simulink model "PMSMwithPSWM"  (R2018a)
settings: Solver=FixedStepDiscrete  StartTime=0.0  StopTime=4  FixedStep=1e-6  RelTol=1e-3
libraries: powerlib x28, simulink x6, powerlib_meascontrol x1
settings Model: Creator=user  LastModifiedBy=Administrator

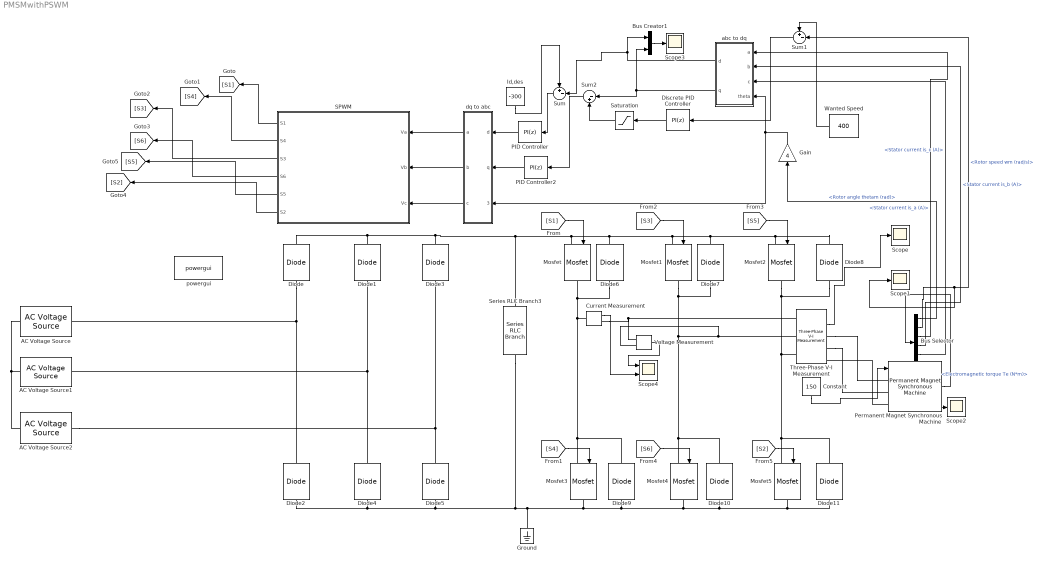
== system PMSMwithPSWM ==
  AC Voltage Source : powerlib/Electrical Sources/AC Voltage Source  Amplitude=230  Phase=0  Frequency=50  SampleTime=0  Measurements=None  BusType=swing  Pref=10e3  Qref=0  Qmin=-inf  Qmax=+inf
  AC Voltage Source1 : powerlib/Electrical Sources/AC Voltage Source  Amplitude=230  Phase=120  Frequency=50  SampleTime=0  Measurements=None  BusType=swing  Pref=10e3  Qref=0  Qmin=-inf  Qmax=+inf
  AC Voltage Source2 : powerlib/Electrical Sources/AC Voltage Source  Amplitude=230  Phase=240  Frequency=50  SampleTime=0  Measurements=None  BusType=swing  Pref=10e3  Qref=0  Qmin=-inf  Qmax=+inf
  Bus Creator1 : BusCreator  Inputs=2
  Bus Selector : BusSelector  OutputSignals=Rotor angle thetam (rad),Rotor speed wm (rad/s),Stator current is_a (A),Stator current is_b (A),Stator current is_c (A),Electromagnetic torque Te (N*m)
  Constant : Constant  Value=150
  Current Measurement : powerlib/Measurements/Current Measurement  PhasorSimulation=off  OutputType=Complex  PSBequivalent=0
  Diode{,1..5} (6 alike) : powerlib/Power Electronics/Diode  Ron=0.02  Lon=0  Vf=0.8  IC=0  UseSnubber=0  Rs=500  Cs=250e-9  Measurements=off
  Diode{6..11} (6 alike) : powerlib/Power Electronics/Diode  Ron=0.001  Lon=0  Vf=0.8  IC=0  UseSnubber=0  Rs=500  Cs=250e-9  Measurements=off
  Discrete PID Controller : simulink/Continuous/PID Controller  Controller=PI  TimeDomain=Discrete-time  SampleTime=-1  IntegratorMethod=Forward Euler  FilterMethod=Forward Euler  Form=Parallel  UseFilter=on  ControllerParametersSource=internal  P=800  I=1  D=0  N=100  InitialConditionSource=internal  InitialConditionForIntegrator=0  InitialConditionForFilter=0  ExternalReset=none  LimitOutput=off  UpperSaturationLimit=inf  LowerSaturationLimit=-inf  LinearizeAsGain=off  AntiWindupMode=none  Kb=1  TrackingMode=off  Kt=1  PParamMin=[]  PParamMax=[]  IParamMin=[]  IParamMax=[]  DParamMin=[]  DParamMax=[]  NParamMin=[]  NParamMax=[]  KbParamMin=[]  KbParamMax=[]  KtParamMin=[]  KtParamMax=[]  POutMin=[]  POutMax=[]  IOutMin=[]  IOutMax=[]  DOutMin=[]  DOutMax=[]  NOutMin=[]  NOutMax=[]  KbOutMin=[]  KbOutMax=[]  KtOutMin=[]  KtOutMax=[]  IntegratorOutMin=[]  IntegratorOutMax=[]  FilterOutMin=[]  FilterOutMax=[]  SumOutMin=[]  SumOutMax=[]  SumI1OutMin=[]  SumI1OutMax=[]  SumI2OutMin=[]  SumI2OutMax=[]  SumI3OutMin=[]  SumI3OutMax=[]  SumDOutMin=[]  SumDOutMax=[]  SaturationOutMin=[]  SaturationOutMax=[]  IntegratorContinuousStateAttributes=''  IntegratorStateMustResolveToSignalObject=off  IntegratorRTWStateStorageClass=Auto  FilterContinuousStateAttributes=''  FilterStateMustResolveToSignalObject=off  FilterRTWStateStorageClass=Auto  DifferentiatorICPrevScaledInput=0  DifferentiatorOutMin=[]  DifferentiatorOutMax=[]  FilterDiffOutCoefMin=[]  FilterDiffOutCoefMax=[]  SumDenOutMin=[]  SumDenOutMax=[]  SumNumOutMin=[]  SumNumOutMax=[]  ReciprocalOutMin=[]  ReciprocalOutMax=[]  DivideOutMin=[]  DivideOutMax=[]  TunerSelectOption=Transfer Function Based (PID Tuner App)
  Gain : Gain  Gain=4
  Ground : powerlib/Elements/Ground  LConnTagsString=a
  Id,des : Constant  Value=-300
  Mosfet{,1..5} (6 alike) : powerlib/Power Electronics/Mosfet  Ron=0.1  Lon=0  Rd=0.01  Vfd=0  IC=0  Rs=1e5  Cs=inf  Measurements=off
  PID Controller : simulink/Continuous/PID Controller  Controller=PI  TimeDomain=Discrete-time  SampleTime=-1  IntegratorMethod=Forward Euler  FilterMethod=Forward Euler  Form=Parallel  UseFilter=on  ControllerParametersSource=internal  P=300  I=40  D=0  N=100  InitialConditionSource=internal  InitialConditionForIntegrator=0  InitialConditionForFilter=0  ExternalReset=none  LimitOutput=off  UpperSaturationLimit=inf  LowerSaturationLimit=-inf  LinearizeAsGain=on  AntiWindupMode=none  Kb=1  TrackingMode=off  Kt=1  PParamMin=[]  PParamMax=[]  IParamMin=[]  IParamMax=[]  DParamMin=[]  DParamMax=[]  NParamMin=[]  NParamMax=[]  KbParamMin=[]  KbParamMax=[]  KtParamMin=[]  KtParamMax=[]  POutMin=[]  POutMax=[]  IOutMin=[]  IOutMax=[]  DOutMin=[]  DOutMax=[]  NOutMin=[]  NOutMax=[]  KbOutMin=[]  KbOutMax=[]  KtOutMin=[]  KtOutMax=[]  IntegratorOutMin=[]  IntegratorOutMax=[]  FilterOutMin=[]  FilterOutMax=[]  SumOutMin=[]  SumOutMax=[]  SumI1OutMin=[]  SumI1OutMax=[]  SumI2OutMin=[]  SumI2OutMax=[]  SumI3OutMin=[]  SumI3OutMax=[]  SumDOutMin=[]  SumDOutMax=[]  SaturationOutMin=[]  SaturationOutMax=[]  IntegratorContinuousStateAttributes=''  IntegratorStateMustResolveToSignalObject=off  IntegratorRTWStateStorageClass=Auto  FilterContinuousStateAttributes=''  FilterStateMustResolveToSignalObject=off  FilterRTWStateStorageClass=Auto  DifferentiatorICPrevScaledInput=0  DifferentiatorOutMin=[]  DifferentiatorOutMax=[]  FilterDiffOutCoefMin=[]  FilterDiffOutCoefMax=[]  SumDenOutMin=[]  SumDenOutMax=[]  SumNumOutMin=[]  SumNumOutMax=[]  ReciprocalOutMin=[]  ReciprocalOutMax=[]  DivideOutMin=[]  DivideOutMax=[]  TunerSelectOption=Transfer Function Based (PID Tuner App)
  PID Controller2 : simulink/Continuous/PID Controller  Controller=PI  TimeDomain=Discrete-time  SampleTime=-1  IntegratorMethod=Forward Euler  FilterMethod=Forward Euler  Form=Parallel  UseFilter=on  ControllerParametersSource=internal  P=300  I=40  D=0  N=100  InitialConditionSource=internal  InitialConditionForIntegrator=0  InitialConditionForFilter=0  ExternalReset=none  LimitOutput=off  UpperSaturationLimit=inf  LowerSaturationLimit=-inf  LinearizeAsGain=on  AntiWindupMode=none  Kb=1  TrackingMode=off  Kt=1  PParamMin=[]  PParamMax=[]  IParamMin=[]  IParamMax=[]  DParamMin=[]  DParamMax=[]  NParamMin=[]  NParamMax=[]  KbParamMin=[]  KbParamMax=[]  KtParamMin=[]  KtParamMax=[]  POutMin=[]  POutMax=[]  IOutMin=[]  IOutMax=[]  DOutMin=[]  DOutMax=[]  NOutMin=[]  NOutMax=[]  KbOutMin=[]  KbOutMax=[]  KtOutMin=[]  KtOutMax=[]  IntegratorOutMin=[]  IntegratorOutMax=[]  FilterOutMin=[]  FilterOutMax=[]  SumOutMin=[]  SumOutMax=[]  SumI1OutMin=[]  SumI1OutMax=[]  SumI2OutMin=[]  SumI2OutMax=[]  SumI3OutMin=[]  SumI3OutMax=[]  SumDOutMin=[]  SumDOutMax=[]  SaturationOutMin=[]  SaturationOutMax=[]  IntegratorContinuousStateAttributes=''  IntegratorStateMustResolveToSignalObject=off  IntegratorRTWStateStorageClass=Auto  FilterContinuousStateAttributes=''  FilterStateMustResolveToSignalObject=off  FilterRTWStateStorageClass=Auto  DifferentiatorICPrevScaledInput=0  DifferentiatorOutMin=[]  DifferentiatorOutMax=[]  FilterDiffOutCoefMin=[]  FilterDiffOutCoefMax=[]  SumDenOutMin=[]  SumDenOutMax=[]  SumNumOutMin=[]  SumNumOutMax=[]  ReciprocalOutMin=[]  ReciprocalOutMax=[]  DivideOutMin=[]  DivideOutMax=[]  TunerSelectOption=Transfer Function Based (PID Tuner App)
  Permanent Magnet Synchronous Machine : powerlib/Machines/Permanent Magnet Synchronous Machine  NbPhases=3  FluxDistribution=Sinusoidal  RotorType=Round  MechanicalLoad=Torque Tm  PresetModel=No  ShowDetailedParameters=on  MeasurementBus=off  Resistance=0.05  Inductance=8.5e-3  dqInductances=[8.5e-3,8.5e-3]  La=0.0005  MachineConstant=Flux linkage established by magnets (V.s)  Flux=0.2  VoltageCst=145.1039  TorqueCst=1.2  Flat=120  Mechanical=[0.1 0.000303448 4]  PolePairs=4  InitialConditions=[10,0, 0.5,0.5]  InitialConditions5ph=[0 0 0 0 0 0]  TsPowergui=0  TsBlock=-1  RefAngle=90 degrees behind phase A axis (modified Park)
      settings: SourceProductName=Simscape Power Systems
  SPWM : Subsystem
  Saturation : Saturate  UpperLimit=270  LowerLimit=-270  LinearizeAsGain=off
  Scope{,1..3} (4 alike) : Scope
  Scope4 : Scope  NumInputPorts=2
  Series RLC Branch3 : powerlib/Elements/Series RLC Branch  LConnTagsString=__new0  RConnTagsString=__new0  BranchType=C  Resistance=1  Inductance=1e-3  SetiL0=off  InitialCurrent=0  Capacitance=0.1  Setx0=off  InitialVoltage=0  Measurements=None
  Sum : Sum  Inputs=+-|
  Sum1 : Sum  Inputs=+-|
  Sum2 : Sum  Inputs=|-+
  Three-Phase V-I Measurement : powerlib/Measurements/Three-Phase V-I Measurement  VoltageMeasurement=phase-to-phase  SetLabelV=off  LabelV=Vabc  Vpu=off  VpuLL=off  CurrentMeasurement=yes  SetLabelI=off  LabelI=Iabc  Ipu=off  Pbase=100e6  Vbase=500e3  OutputType=Complex  PhasorSimulation=off  PSBequivalent=0
  Voltage Measurement : powerlib/Measurements/Voltage Measurement  PhasorSimulation=off  OutputType=Complex  PSBequivalent=0
  Wanted Speed : Constant  Value=400
  abc to dq : MATLAB Function  TreatAsAtomicUnit=on
  dq to abc : MATLAB Function  TreatAsAtomicUnit=on
  powergui : powerlib/powergui  Priority=1  SimulationMode=Discrete  SampleTime=1e-6  frequency=60  Iterations=50  frequencyindice=50  Pbase=100e6  ErrMax=1e-4  UnitsV=kV  UnitsW=MW  buscounter=0  FunctionMessages=off  echomessages=off  EnableUseOfTLC=off  CurrentSourceSwitches=off  DisableSnubberDevices=off  DisableRonSwitches=off  DisableVfSwitches=off  DisplayEquations=off  SolverType=Tustin/Backward Euler (TBE)  Interpol=off  ExternalGateDelay=off  methode=off  Ts=100  x0status=blocks  SPID=off  SwTol=0  HookPort=off  RestoreLinks=warning  ResistiveCurrentMeasurement=off  Frange=[0:2:500]  Ylog=off  Xlog=on  ShowGrid=off  save=off  variable=ZData  structure=0  ZoomFFT=off  StartTime=0.0  cycles=1  DisplayStyle=1  fundamental=60  FreqAxis=off  MaxFrequency=1000  frequencyindicesteady=1  RmsSteady=1  display=off
  wires:
  Permanent Magnet Synchronous Machine/1 -> Bus Selector/1
  Bus Selector/1 -> Gain/1  "<Rotor angle thetam (rad)>"
  Id,des/1 -> Sum/1
  Sum/1 -> PID Controller/1
  abc to dq/2(q) -> Sum2/1, Bus Creator1/2
  Sum2/1 -> PID Controller2/1
  Bus Selector/2 -> Sum1/2, Scope1/1  "<Rotor speed wm (rad/s)>"
  Wanted Speed/1 -> Sum1/1
  Sum1/1 -> Discrete PID Controller/1
  Discrete PID Controller/1 -> Saturation/1
  Bus Selector/3 -> abc to dq/1(a)  "<Stator current is_a (A)>"
  Bus Selector/4 -> abc to dq/2(b)  "<Stator current is_b (A)>"
  Bus Selector/5 -> abc to dq/3(c)  "<Stator current is_c (A)>"
  PID Controller/1 -> dq to abc/1(d)
  PID Controller2/1 -> dq to abc/2(q)
  dq to abc/2(b) -> SPWM/2(Vb)
  dq to abc/1(a) -> SPWM/1(Va)
  dq to abc/3(c) -> SPWM/3(Vc)
  SPWM/1(S1) -> [S1]
  SPWM/2(S4) -> [S4]
  SPWM/3(S3) -> [S3]
  SPWM/4(S6) -> [S6]
  SPWM/6(S2) -> [S2]
  SPWM/5(S5) -> [S5]
  [S1] -> Mosfet/1
  [S4] -> Mosfet3/1
  [S3] -> Mosfet1/1
  [S5] -> Mosfet2/1
  [S6] -> Mosfet4/1
  [S2] -> Mosfet5/1
  Constant/1 -> Permanent Magnet Synchronous Machine/1
  Saturation/1 -> Sum2/2
  Gain/1 -> dq to abc/3(theta), abc to dq/4(theta)
  Bus Selector/6 -> Scope2/1  "<Electromagnetic torque Te (N*m)>"
  abc to dq/1(d) -> Bus Creator1/1, Sum/2
  Bus Creator1/1 -> Scope3/1
  Voltage Measurement/1 -> Scope4/1
  Current Measurement/1 -> Scope4/2
  Three-Phase V-I Measurement/2 -> Scope/1
  connections:
  Diode4/RConn1 -- AC Voltage Source1/RConn1 -- Diode1/LConn1
  Diode5/RConn1 -- AC Voltage Source2/RConn1 -- Diode3/LConn1
  Diode/RConn1 -- Diode8/RConn1 -- Mosfet2/LConn1 -- Diode7/RConn1 -- Mosfet1/LConn1 -- Diode6/RConn1 -- Mosfet/LConn1 -- Series RLC Branch3/LConn1 -- Diode3/RConn1 -- Diode1/RConn1
  AC Voltage Source/LConn1 -- AC Voltage Source2/LConn1 -- AC Voltage Source1/LConn1
  Diode/LConn1 -- AC Voltage Source/RConn1 -- Diode2/RConn1
  Mosfet1/RConn1 -- Diode7/LConn1 -- Voltage Measurement/LConn2 -- Three-Phase V-I Measurement/LConn2 -- Diode10/RConn1 -- Mosfet4/LConn1
  Mosfet3/LConn1 -- Diode9/RConn1 -- Diode6/LConn1 -- Mosfet/RConn1 -- Current Measurement/LConn1
  Mosfet2/RConn1 -- Diode8/LConn1 -- Diode11/RConn1 -- Mosfet5/LConn1 -- Three-Phase V-I Measurement/LConn3
  Diode9/LConn1 -- Ground/LConn1 -- Diode2/LConn1 -- Diode4/LConn1 -- Diode5/LConn1 -- Series RLC Branch3/RConn1 -- Mosfet3/RConn1 -- Diode11/LConn1 -- Mosfet5/RConn1 -- Diode10/LConn1 -- Mosfet4/RConn1
  Three-Phase V-I Measurement/RConn1 -- Permanent Magnet Synchronous Machine/LConn1
  Three-Phase V-I Measurement/RConn2 -- Permanent Magnet Synchronous Machine/LConn2
  Permanent Magnet Synchronous Machine/LConn3 -- Three-Phase V-I Measurement/RConn3
  Three-Phase V-I Measurement/LConn1 -- Current Measurement/RConn1 -- Voltage Measurement/LConn1

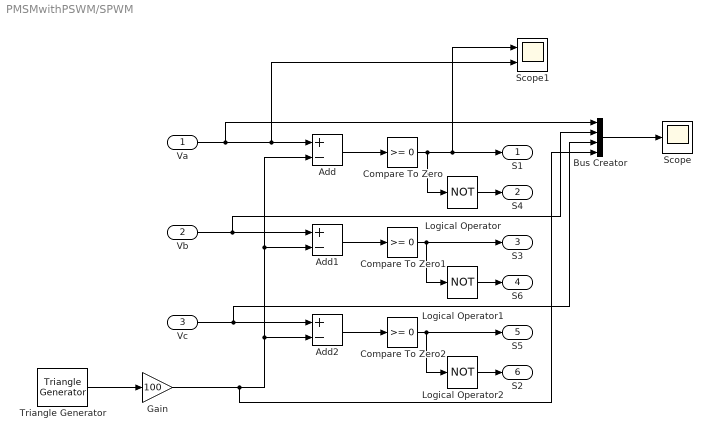
== system PMSMwithPSWM/SPWM ==
  Va : Inport
  Vb : Inport  Port=2
  Vc : Inport  Port=3
  Add : Sum  Inputs=+-
  Add1 : Sum  Inputs=+-
  Add2 : Sum  Inputs=+-
  Bus Creator : BusCreator  Inputs=4
  Compare To Zero : simulink/Logic and Bit Operations/Compare To Zero  relop=>=  OutDataTypeStr=boolean
  Compare To Zero1 : simulink/Logic and Bit Operations/Compare To Zero  relop=>=  OutDataTypeStr=boolean
  Compare To Zero2 : simulink/Logic and Bit Operations/Compare To Zero  relop=>=  OutDataTypeStr=boolean
  Gain : Gain  Gain=100
  Logical Operator : Logic  Operator=NOT  AllPortsSameDT=off  OutDataTypeStr=boolean
  Logical Operator1 : Logic  Operator=NOT  AllPortsSameDT=off  OutDataTypeStr=boolean
  Logical Operator2 : Logic  Operator=NOT  AllPortsSameDT=off  OutDataTypeStr=boolean
  Scope : Scope
  Scope1 : Scope  NumInputPorts=2
  Triangle Generator : powerlib_meascontrol/Pulse & Signal Generators/Triangle Generator  Freq=1e4  Phase=90  Ts=0
  S1 : Outport
  S4 : Outport  Port=2
  S3 : Outport  Port=3
  S6 : Outport  Port=4
  S5 : Outport  Port=5
  S2 : Outport  Port=6
  wires:
  Compare To Zero2/1 -> S5/1, Logical Operator2/1
  Vc/1 -> Bus Creator/3, Add2/1
  Compare To Zero1/1 -> S3/1, Logical Operator1/1
  Bus Creator/1 -> Scope/1
  Add1/1 -> Compare To Zero1/1
  Logical Operator1/1 -> S6/1
  Logical Operator2/1 -> S2/1
  Vb/1 -> Bus Creator/2, Add1/1
  Va/1 -> Bus Creator/1, Scope1/2, Add/1
  Triangle Generator/1 -> Gain/1
  Add/1 -> Compare To Zero/1
  Compare To Zero/1 -> Logical Operator/1, S1/1, Scope1/1
  Add2/1 -> Compare To Zero2/1
  Logical Operator/1 -> S4/1
  Gain/1 -> Bus Creator/4, Add1/2, Add/2, Add2/2

== matlab function PMSMwithPSWM/dq to abc ==
  data: d input; a output; q input; theta input; b output; c output
function [a,b,c] = fcn(d,q,theta)
a = d* sin(theta)+ q* cos(theta) ;

b = d * sin(theta-2*pi/3) + q*cos(theta-2*pi/3);

c = d*sin(theta+2*pi/3)+q*cos(theta+2*pi/3);

== matlab function PMSMwithPSWM/abc to dq ==
  data: a input; d output; b input; c input; theta input; q output
function [d,q] = fcn(a,b,c,theta)
d = a * sin(theta) + b*sin(theta-2*pi/3)+c*sin(theta+2*pi/3);
q = a* cos(theta)+ b* cos(theta-2*pi/3)+c*cos(theta+2*pi/3);
